simulink model "inga2"  (R2013a)
settings: Solver=ode45  StartTime=0.0  StopTime=100  MaxStep=0.1  RelTol=1e-3
settings Model: Creator=Kinga  LastModifiedBy=rudi
settings DataIOCC: SignalLoggingSaveFormat=ModelDataLogs
settings DebuggingCC: UnderspecifiedInitializationDetection=Simplified  MultiTaskDSMMsg=warning  MultiTaskCondExecSysMsg=none  StateNameClashWarn=none  StrictBusMsg=ErrorOnBusTreatedAsVector
settings RTWCC: IncludeERTFirstTime=on
settings GRTTargetCC: CodeReplacementLibrary=None  CPPClassGenCompliant=on

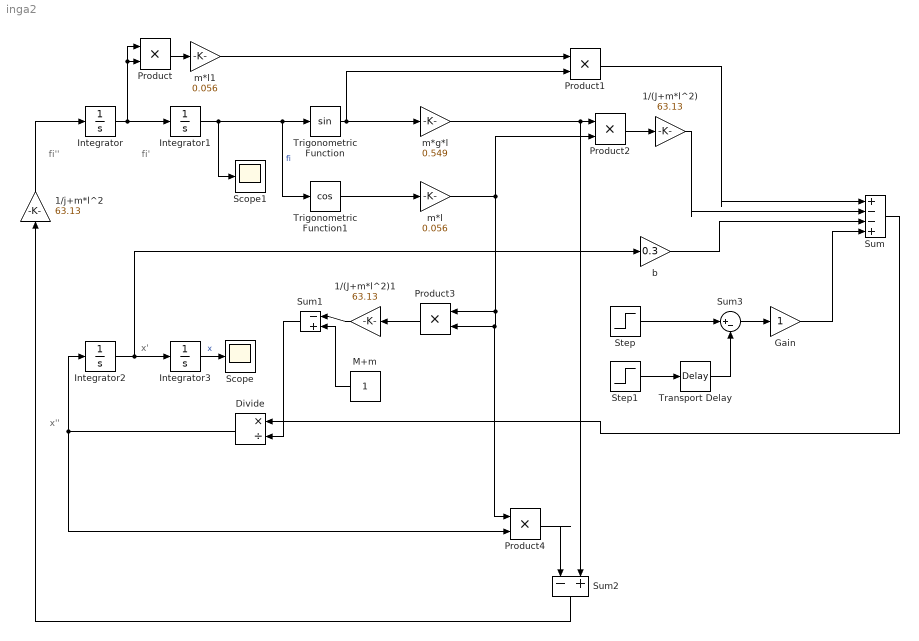
== system inga2 ==
  note: x''
  note: x'
  note: fi''
  note: fi'
  1/(J+m*l^2) : Gain  Gain=63.13
  1/(J+m*l^2)1 : Gain  Gain=63.13
  1/j+m*l^2 : Gain  Gain=63.13
  Divide : Product  Inputs=*/
  Gain : Gain
  Integrator{,1..3} (4 alike) : Integrator
  M+m : Constant
  Product{,1..4} (5 alike) : Product
  Scope : Scope
  Scope1 : Scope
      settings: TimeRange=50
  Step : Step  SampleTime=0
  Step1 : Step  Time=2  SampleTime=0
  Sum : Sum  Inputs=|+--+
  Sum1 : Sum  Inputs=|-+
  Sum2 : Sum  Inputs=|-+
  Sum3 : Sum  Inputs=|+-
  Transport Delay : TransportDelay
  Trigonometric Function : Trigonometry
  Trigonometric Function1 : Trigonometry  Operator=cos
  b : Gain  Gain=0.3
  m*g*l : Gain  Gain=0.549
  m*l : Gain  Gain=0.056
  m*l1 : Gain  Gain=0.056
  wires:
  Integrator/1 -> Integrator1/1, Product/1, Product/2
  Integrator2/1 -> b/1, Integrator3/1
  Integrator1/1 -> Trigonometric Function1/1, Trigonometric Function/1, Scope1/1  "fi"
  Trigonometric Function/1 -> Product1/2, m*g*l/1
  Trigonometric Function1/1 -> m*l/1
  Product/1 -> m*l1/1
  m*l1/1 -> Product1/1
  m*g*l/1 -> Sum2/2, Product2/1
  m*l/1 -> Product3/1, Product3/2, Product4/1, Product2/2
  Product2/1 -> 1/(J+m*l^2)/1
  Product1/1 -> Sum/1
  1/(J+m*l^2)/1 -> Sum/2
  b/1 -> Sum/3
  Product3/1 -> 1/(J+m*l^2)1/1
  M+m/1 -> Sum1/2
  1/(J+m*l^2)1/1 -> Sum1/1
  Divide/1 -> Product4/2, Integrator2/1
  1/j+m*l^2/1 -> Integrator/1
  Product4/1 -> Sum2/1
  Sum2/1 -> 1/j+m*l^2/1
  Integrator3/1 -> Scope/1  "x"
  Sum1/1 -> Divide/2
  Sum/1 -> Divide/1
  Step1/1 -> Transport Delay/1
  Step/1 -> Sum3/1
  Transport Delay/1 -> Sum3/2
  Sum3/1 -> Gain/1
  Gain/1 -> Sum/4
